simulink model "SAC_BSFC_Simulink"  (R2024b)
settings: Solver=VariableStepAuto  StartTime=0.0  StopTime=5  RelTol=1e-3
values from neighbouring files (symbols this model uses):
  BSFC = [0 0 0 0 0 0 0 0 0 0 0 0 ... (2442 elements, 37x66)]    [BSFC_LuT.mat]
  ScalerOut_range = [4.67113400e-01 3.79188137e-06 1.99107205e-09 1.76146956e-01]    [SACsim_params.m]
  ScalerOutMax = [8.17552600e-01 3.79204100e-06 1.99143300e-09 1.02194086e-01]    [SACsim_params.m]
  ScalerOutMin = [3.5043920e-01 1.5963114e-10 3.6094947e-13 -7.3952870e-02]    [SACsim_params.m]
  Tice_bp_BSFC = [0 5 10 15 20 25 30 35 40 45 50 55 ... (66 elements, 1x66)]    [BSFC_LuT.mat]
  wice_bp_BSFC = [0 13.08996939 26.1799387799 39.2699081699 52.3598775598 65.4498469498 78.5398163397 91.6297857297 104.71975512 117.80972451 130.8996939 143.98966329 ... (37 elements, 1x37)]    [BSFC_LuT.mat]
undefined symbols (not defined in the file or in its folder): a1, a2, Eng_pwr_opt_list, float32, NOx_ref, ScalerSACMax, ScalerSACMin, SoC_ref, W_list
libraries: pycoexlib x1, rllib x1
settings Model: Creator=fjcub  LastModifiedBy=fjcub

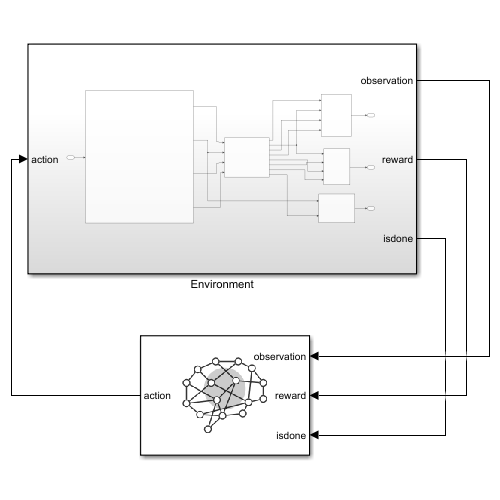
[thumbnail: Simulink's stored preview of the top-level diagram]
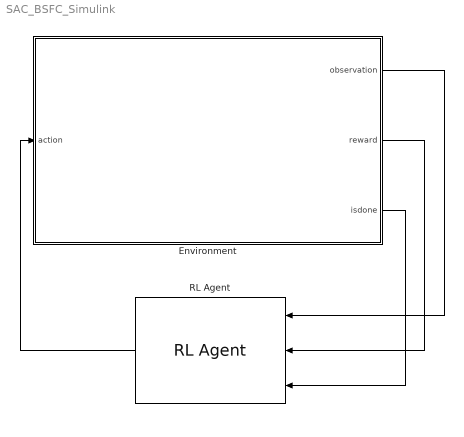
== system SAC_BSFC_Simulink ==
  Environment : Subsystem
  RL Agent : rllib/RL Agent  Agent=agent  ExternalActionAsInput=off  ProvideLastAction=off  ProvideCumRwd=off  TreatAsDirectFeedthrough=on  UseStrictObservationDataTypes=off
  wires:
  Environment/1(observation) -> RL Agent/1
  Environment/2(reward) -> RL Agent/2
  Environment/3(isdone) -> RL Agent/3
  RL Agent/1 -> Environment/1(action)

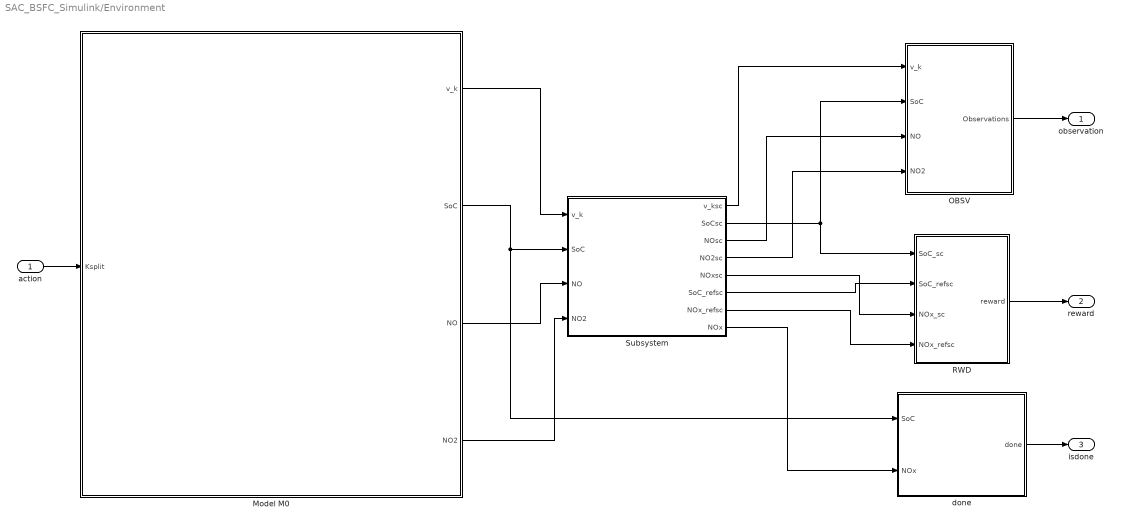
== system SAC_BSFC_Simulink/Environment ==
  action : Inport
  Model M0 : Subsystem
  OBSV : Subsystem
  RWD : Subsystem
  Subsystem : Subsystem
  done : Subsystem
  observation : Outport
  reward : Outport  Port=2
  isdone : Outport  Port=3
  wires:
  OBSV/1(Observations) -> observation/1
  action/1 -> Model M0/1(Ksplit)
  RWD/1(reward) -> reward/1
  done/1(done) -> isdone/1
  Model M0/1(v_k) -> Subsystem/1(v_k)
  Model M0/2(SoC) -> done/1(SoC), Subsystem/2(SoC)
  Model M0/3(NO) -> Subsystem/3(NO)
  Model M0/4(NO2) -> Subsystem/4(NO2)
  Subsystem/8(NOx) -> done/2(NOx)
  Subsystem/7(NOx_refsc) -> RWD/4(NOx_refsc)
  Subsystem/5(NOxsc) -> RWD/3(NOx_sc)
  Subsystem/6(SoC_refsc) -> RWD/2(SoC_refsc)
  Subsystem/2(SoCsc) -> OBSV/2(SoC), RWD/1(SoC_sc)
  Subsystem/1(v_ksc) -> OBSV/1(v_k)
  Subsystem/3(NOsc) -> OBSV/3(NO)
  Subsystem/4(NO2sc) -> OBSV/4(NO2)

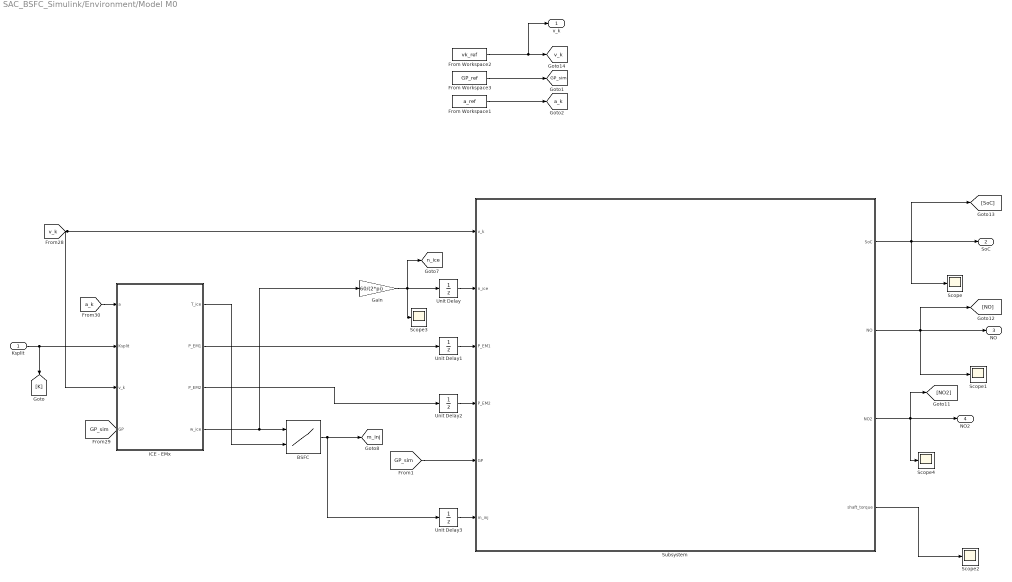
== system SAC_BSFC_Simulink/Environment/Model M0 ==
  Ksplit : Inport
  BSFC : Lookup_n-D  BreakpointsForDimension1=wice_bp_BSFC  BreakpointsForDimension2=Tice_bp_BSFC  Table=BSFC  InternalRulePriority=Speed  RndMeth=Simplest
      settings: InputPortMap=u0,u1
  From Workspace1 : FromWorkspace  VariableName=a_ref  SampleTime=1
  From Workspace2 : FromWorkspace  VariableName=vk_ref  SampleTime=1
  From Workspace3 : FromWorkspace  VariableName=GP_ref  SampleTime=1
  Gain : Gain  Gain=60/(2*pi)
  ICE - EMx : Subsystem
  Scope{,1..4} (5 alike) : Scope
  Subsystem : Subsystem
  Unit Delay{,1..3} (4 alike) : UnitDelay  SampleTime=-1  HasFrameUpgradeWarning=on
  v_k : Outport
  SoC : Outport  Port=2
  NO : Outport  Port=3
  NO2 : Outport  Port=4
  tag scope: GP_sim=global, a_k=global, m_inj=global, n_ice=global, v_k=global
  wires:
  From Workspace1/1 -> [a_k]
  From Workspace3/1 -> [GP_sim]
  From Workspace2/1 -> v_k/1, [v_k]
  Gain/1 -> Unit Delay/1, [n_ice], Scope3/1
  ICE - EMx/1(T_ice) -> BSFC/2
  Subsystem/4(shaft_torque) -> Scope2/1
  [GP_sim] -> ICE - EMx/4(GP)
  Subsystem/2(NO) -> Scope1/1, NO/1, [NO]
  [v_k] -> ICE - EMx/3(v_k), Subsystem/1(v_k)
  ICE - EMx/3(P_EM2) -> Unit Delay2/1
  Subsystem/1(SoC) -> Scope/1, SoC/1, [SoC]
  ICE - EMx/2(P_EM1) -> Unit Delay1/1
  [a_k] -> ICE - EMx/1(a)
  BSFC/1 -> Unit Delay3/1, [m_inj]
  [GP_sim] -> Subsystem/5(GP)
  ICE - EMx/4(w_ice) -> Gain/1, BSFC/1
  Ksplit/1 -> ICE - EMx/2(Ksplit), [K]
  Subsystem/3(NO2) -> [NO2], NO2/1, Scope4/1
  Unit Delay/1 -> Subsystem/2(n_ice)
  Unit Delay1/1 -> Subsystem/3(P_EM1)
  Unit Delay2/1 -> Subsystem/4(P_EM2)
  Unit Delay3/1 -> Subsystem/6(m_inj)

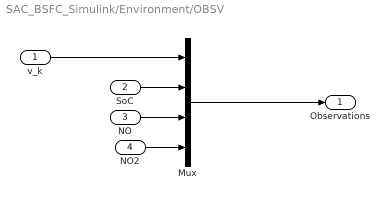
== system SAC_BSFC_Simulink/Environment/OBSV ==
  v_k : Inport
  SoC : Inport  Port=2
  NO : Inport  Port=3
  NO2 : Inport  Port=4
  Mux : Mux
  Observations : Outport
  wires:
  v_k/1 -> Mux/1
  SoC/1 -> Mux/2
  NO2/1 -> Mux/4
  NO/1 -> Mux/3
  Mux/1 -> Observations/1

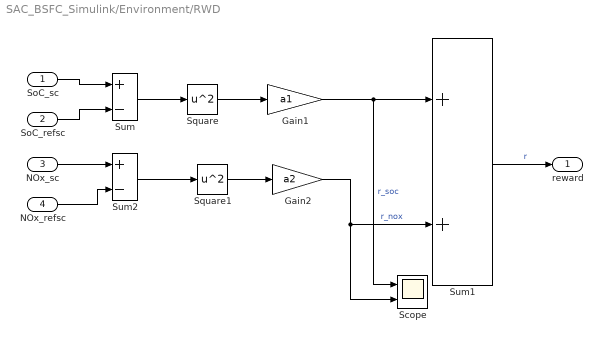
== system SAC_BSFC_Simulink/Environment/RWD ==
  SoC_sc : Inport
  SoC_refsc : Inport  Port=2
  NOx_sc : Inport  Port=3
  NOx_refsc : Inport  Port=4
  Gain1 : Gain  Gain=a1
  Gain2 : Gain  Gain=a2
  Scope : Scope  NumInputPorts=2
  Square : Math  Operator=square
  Square1 : Math  Operator=square
  Sum : Sum  Inputs=+-
  Sum1 : Sum
  Sum2 : Sum  Inputs=+-
  reward : Outport
  wires:
  Sum1/1 -> reward/1  "r"
  Sum/1 -> Square/1
  Square1/1 -> Gain2/1
  Sum2/1 -> Square1/1
  Gain1/1 -> Sum1/1, Scope/1  "r_soc"
  Gain2/1 -> Scope/2, Sum1/2  "r_nox"
  Square/1 -> Gain1/1
  SoC_sc/1 -> Sum/1
  SoC_refsc/1 -> Sum/2
  NOx_sc/1 -> Sum2/1
  NOx_refsc/1 -> Sum2/2

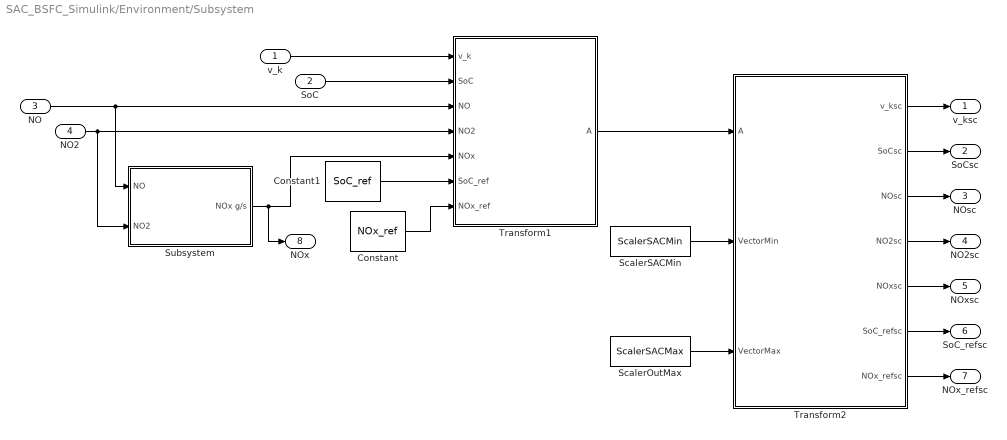
== system SAC_BSFC_Simulink/Environment/Subsystem ==
  v_k : Inport
  SoC : Inport  Port=2
  NO : Inport  Port=3
  NO2 : Inport  Port=4
  Constant : Constant  Value=NOx_ref
  Constant1 : Constant  Value=SoC_ref
  ScalerOutMax : Constant  Value=ScalerSACMax
  ScalerSACMin : Constant  Value=ScalerSACMin
  Subsystem : Subsystem
  Transform1 : MATLAB Function  TreatAsAtomicUnit=on
  Transform2 : MATLAB Function  TreatAsAtomicUnit=on
  v_ksc : Outport
  SoCsc : Outport  Port=2
  NOsc : Outport  Port=3
  NO2sc : Outport  Port=4
  NOxsc : Outport  Port=5
  SoC_refsc : Outport  Port=6
  NOx_refsc : Outport  Port=7
  NOx : Outport  Port=8
  wires:
  v_k/1 -> Transform1/1(v_k)
  SoC/1 -> Transform1/2(SoC)
  NO/1 -> Transform1/3(NO), Subsystem/1(NO)
  NO2/1 -> Subsystem/2(NO2), Transform1/4(NO2)
  Constant/1 -> Transform1/7(NOx_ref)
  Constant1/1 -> Transform1/6(SoC_ref)
  Subsystem/1(NOx g/s) -> Transform1/5(NOx), NOx/1
  Transform2/7(NOx_refsc) -> NOx_refsc/1
  Transform2/6(SoC_refsc) -> SoC_refsc/1
  Transform2/5(NOxsc) -> NOxsc/1
  Transform2/4(NO2sc) -> NO2sc/1
  Transform2/3(NOsc) -> NOsc/1
  Transform2/2(SoCsc) -> SoCsc/1
  Transform1/1(A) -> Transform2/1(A)
  ScalerSACMin/1 -> Transform2/2(VectorMin)
  ScalerOutMax/1 -> Transform2/3(VectorMax)
  Transform2/1(v_ksc) -> v_ksc/1

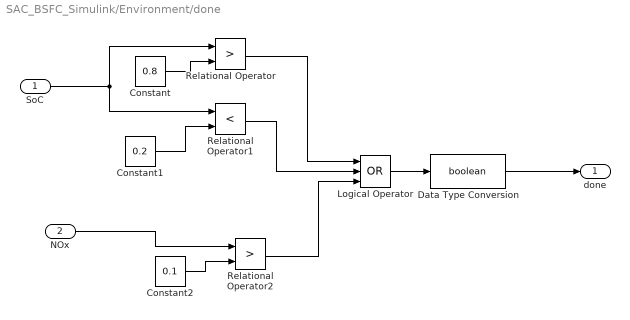
== system SAC_BSFC_Simulink/Environment/done ==
  SoC : Inport
  NOx : Inport  Port=2
  Constant : Constant  Value=0.8
  Constant1 : Constant  Value=0.2
  Constant2 : Constant  Value=0.1
  Data Type Conversion : DataTypeConversion  OutDataTypeStr=boolean  SaturateOnIntegerOverflow=off  RndMeth=Floor
  Logical Operator : Logic  Operator=OR  Inputs=3  AllPortsSameDT=off  OutDataTypeStr=boolean
  Relational Operator : RelationalOperator  Operator=>  OutDataTypeStr=boolean  RndMeth=Simplest  InputSameDT=off
  Relational Operator1 : RelationalOperator  Operator=<  OutDataTypeStr=boolean  RndMeth=Simplest  InputSameDT=off
  Relational Operator2 : RelationalOperator  Operator=>  OutDataTypeStr=boolean  RndMeth=Simplest  InputSameDT=off
  done : Outport
  wires:
  Logical Operator/1 -> Data Type Conversion/1
  Relational Operator/1 -> Logical Operator/1
  Relational Operator1/1 -> Logical Operator/2
  SoC/1 -> Relational Operator1/1, Relational Operator/1
  Constant1/1 -> Relational Operator1/2
  Constant/1 -> Relational Operator/2
  Constant2/1 -> Relational Operator2/2
  NOx/1 -> Relational Operator2/1
  Relational Operator2/1 -> Logical Operator/3
  Data Type Conversion/1 -> done/1

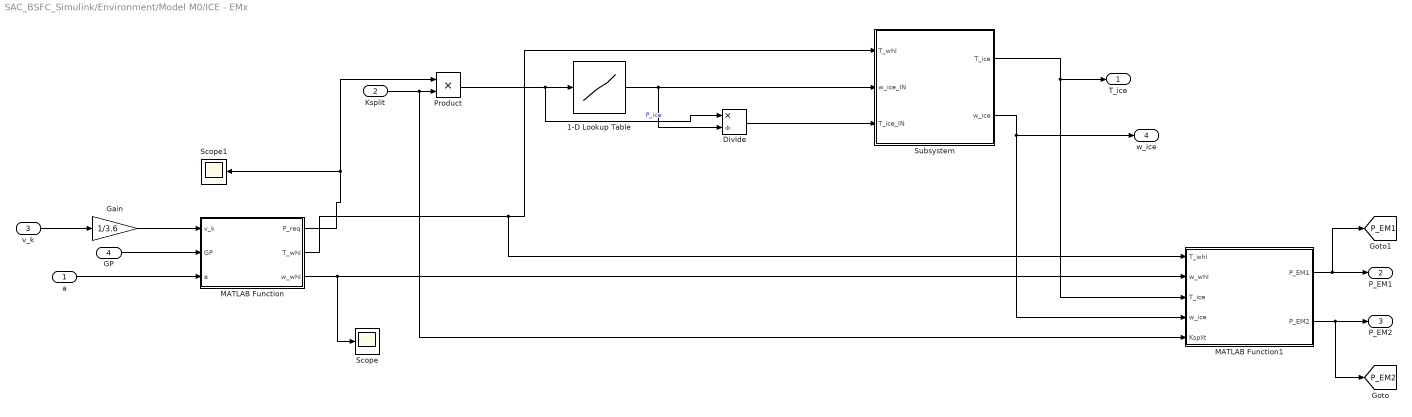
== system SAC_BSFC_Simulink/Environment/Model M0/ICE - EMx ==
  a : Inport
  Ksplit : Inport  Port=2
  v_k : Inport  Port=3
  GP : Inport  Port=4
  1-D Lookup Table : Lookup_n-D  NumberOfTableDimensions=1  BreakpointsForDimension1=Eng_pwr_opt_list  Table=W_list  InternalRulePriority=Speed  RndMeth=Simplest
  Divide : Product  Inputs=*/
  Gain : Gain  Gain=1/3.6
  MATLAB Function : MATLAB Function  TreatAsAtomicUnit=on
  MATLAB Function1 : MATLAB Function  TreatAsAtomicUnit=on
  Product : Product
  Scope : Scope
  Scope1 : Scope
  Subsystem : Subsystem
  T_ice : Outport
  P_EM1 : Outport  Port=2
  P_EM2 : Outport  Port=3
  w_ice : Outport  Port=4
  tag scope: P_EM1=global, P_EM2=global
  wires:
  MATLAB Function1/2(P_EM2) -> [P_EM2], P_EM2/1
  MATLAB Function1/1(P_EM1) -> [P_EM1], P_EM1/1
  MATLAB Function/3(w_whl) -> MATLAB Function1/2(w_whl), Scope/1
  Ksplit/1 -> MATLAB Function1/5(Ksplit), Product/2
  MATLAB Function/1(P_req) -> Product/1, Scope1/1
  GP/1 -> MATLAB Function/2(GP)
  Gain/1 -> MATLAB Function/1(v_k)
  v_k/1 -> Gain/1
  a/1 -> MATLAB Function/3(a)
  Subsystem/1(T_ice) -> T_ice/1, MATLAB Function1/3(T_ice)
  MATLAB Function/2(T_whl) -> MATLAB Function1/1(T_whl), Subsystem/1(T_whl)
  Subsystem/2(w_ice) -> MATLAB Function1/4(w_ice), w_ice/1
  Product/1 -> Divide/1, 1-D Lookup Table/1  "P_ice"
  Divide/1 -> Subsystem/3(T_ice_IN)
  1-D Lookup Table/1 -> Divide/2, Subsystem/2(w_ice_IN)

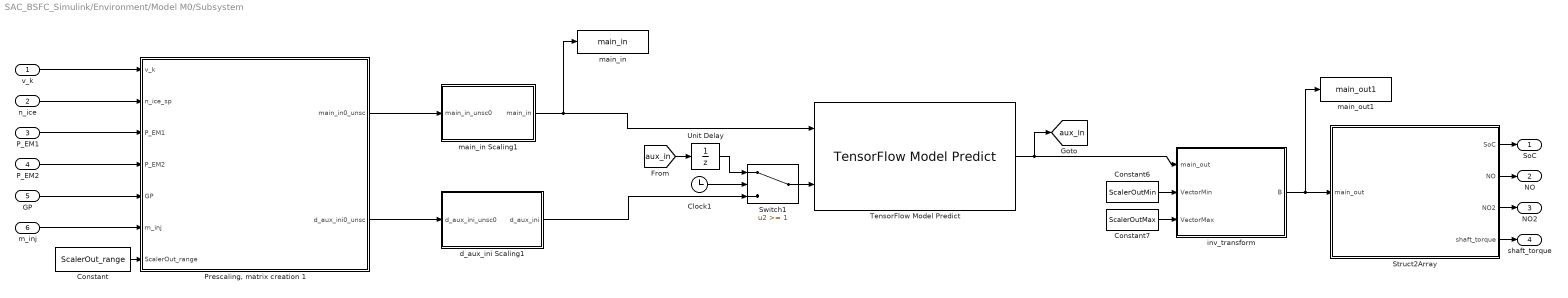
== system SAC_BSFC_Simulink/Environment/Model M0/Subsystem ==
  v_k : Inport
  n_ice : Inport  Port=2
  P_EM1 : Inport  Port=3
  P_EM2 : Inport  Port=4
  GP : Inport  Port=5
  m_inj : Inport  Port=6
  Clock1 : Clock
  Constant : Constant  Value=ScalerOut_range
  Constant6 : Constant  Value=ScalerOutMin
  Constant7 : Constant  Value=ScalerOutMax
  "Prescaling, matrix creation 1" : MATLAB Function  TreatAsAtomicUnit=on
  Struct2Array : MATLAB Function  TreatAsAtomicUnit=on
  Switch1 : Switch  Threshold=1  OutDataTypeStr=double  SaturateOnIntegerOverflow=off  InputSameDT=off
  TensorFlow Model Predict : pycoexlib/TensorFlow Model Predict  ModelFile=C:\Users\fjcub\Documents\UPC\INIREC\CORNET\Models\model.h5  InputTable={ 'main_in', 'float32', '', '3'; 'aux_in', 'float32', '', '3' }  OutputTable={ 'main_out', '', '' }  SampleTime=1  InputDatatypes=float32,float32  InputNumDims=3,3  InputPermutations=[],[]  OutputPermutations=[]  PythonCoexecutionBlockType=TensorFlowModelBlock  VariableOutputMaxSizes=[]
  Unit Delay : UnitDelay  SampleTime=-1  HasFrameUpgradeWarning=on
  d_aux_ini Scaling1 : Subsystem
  inv_transform : MATLAB Function  TreatAsAtomicUnit=on
  main_in : ToWorkspace  VariableName=main_in  SampleTime=1
  main_in Scaling1 : Subsystem
  main_out1 : ToWorkspace  VariableName=main_out1  SampleTime=1
  SoC : Outport
  NO : Outport  Port=2
  NO2 : Outport  Port=3
  shaft_torque : Outport  Port=4
  tag scope: aux_in=global
  wires:
  m_inj/1 -> "Prescaling, matrix creation 1"/6(m_inj)
  P_EM1/1 -> "Prescaling, matrix creation 1"/3(P_EM1)
  TensorFlow Model Predict/1 -> inv_transform/1(main_out), [aux_in]
  inv_transform/1(B) -> main_out1/1, Struct2Array/1(main_out)
  n_ice/1 -> "Prescaling, matrix creation 1"/2(n_ice_sp)
  Struct2Array/3(NO2) -> NO2/1
  Constant/1 -> "Prescaling, matrix creation 1"/7(ScalerOut_range)
  Constant6/1 -> inv_transform/2(VectorMin)
  P_EM2/1 -> "Prescaling, matrix creation 1"/4(P_EM2)
  "Prescaling, matrix creation 1"/1(main_in0_unsc) -> main_in Scaling1/1(main_in_unsc0)
  GP/1 -> "Prescaling, matrix creation 1"/5(GP)
  Struct2Array/2(NO) -> NO/1
  Clock1/1 -> Switch1/2
  Struct2Array/1(SoC) -> SoC/1
  Constant7/1 -> inv_transform/3(VectorMax)
  Struct2Array/4(shaft_torque) -> shaft_torque/1
  "Prescaling, matrix creation 1"/2(d_aux_ini0_unsc) -> d_aux_ini Scaling1/1(d_aux_ini_unsc0)
  main_in Scaling1/1(main_in) -> TensorFlow Model Predict/1, main_in/1
  v_k/1 -> "Prescaling, matrix creation 1"/1(v_k)
  Switch1/1 -> TensorFlow Model Predict/2
  d_aux_ini Scaling1/1(d_aux_ini) -> Switch1/3
  Unit Delay/1 -> Switch1/1
  [aux_in] -> Unit Delay/1

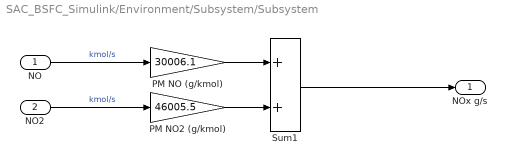
== system SAC_BSFC_Simulink/Environment/Subsystem/Subsystem ==
  NO : Inport
  NO2 : Inport  Port=2
  PM NO (g/kmol) : Gain  Gain=30006.1
  PM NO2 (g/kmol) : Gain  Gain=46005.5
  Sum1 : Sum
  NOx g/s : Outport
  wires:
  PM NO (g/kmol)/1 -> Sum1/1
  PM NO2 (g/kmol)/1 -> Sum1/2
  NO/1 -> PM NO (g/kmol)/1  "kmol/s"
  NO2/1 -> PM NO2 (g/kmol)/1  "kmol/s"
  Sum1/1 -> NOx g/s/1

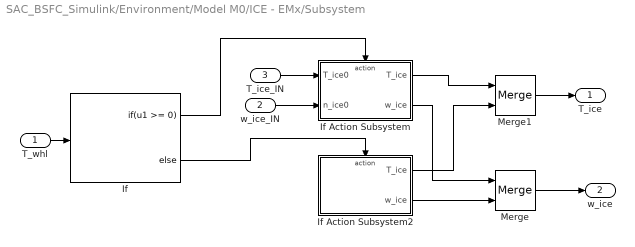
== system SAC_BSFC_Simulink/Environment/Model M0/ICE - EMx/Subsystem ==
  T_whl : Inport
  w_ice_IN : Inport  Port=2
  T_ice_IN : Inport  Port=3
  If : If  IfExpression=u1 >= 0
  If Action Subsystem : Subsystem  TreatAsAtomicUnit=on
  If Action Subsystem2 : Subsystem  TreatAsAtomicUnit=on
  Merge : Merge
  Merge1 : Merge
  T_ice : Outport
  w_ice : Outport  Port=2
  wires:
  T_whl/1 -> If/1
  If/1 -> If Action Subsystem/Action
  If/2 -> If Action Subsystem2/Action
  T_ice_IN/1 -> If Action Subsystem/1(T_ice0)
  w_ice_IN/1 -> If Action Subsystem/2(n_ice0)
  If Action Subsystem/1(T_ice) -> Merge1/1
  If Action Subsystem2/1(T_ice) -> Merge1/2
  If Action Subsystem/2(w_ice) -> Merge/1
  If Action Subsystem2/2(w_ice) -> Merge/2
  Merge/1 -> w_ice/1
  Merge1/1 -> T_ice/1

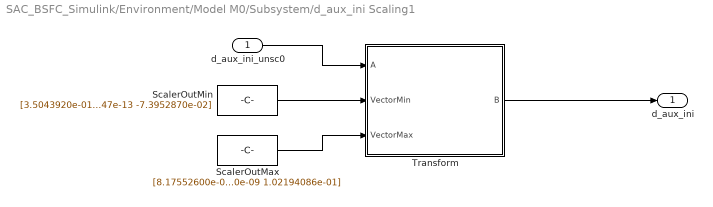
== system SAC_BSFC_Simulink/Environment/Model M0/Subsystem/d_aux_ini Scaling1 ==
  d_aux_ini_unsc0 : Inport
  ScalerOutMax : Constant  Value=[8.17552600e-01 3.79204100e-06 1.99143300e-09 1.02194086e-01]
  ScalerOutMin : Constant  Value=[3.5043920e-01 1.5963114e-10 3.6094947e-13 -7.3952870e-02]
  Transform : MATLAB Function  TreatAsAtomicUnit=on
  d_aux_ini : Outport
  wires:
  d_aux_ini_unsc0/1 -> Transform/1(A)
  ScalerOutMin/1 -> Transform/2(VectorMin)
  ScalerOutMax/1 -> Transform/3(VectorMax)
  Transform/1(B) -> d_aux_ini/1

== system SAC_BSFC_Simulink/Environment/Model M0/Subsystem/main_in Scaling1 ==
  main_in_unsc0 : Inport
  ScalerInMax : Constant  Value=[1.5060300e+02; 2.8380360e+03; 8.5859970e+00; 5.1123200e+01; 4.4160643e+00; 1.2493309e+00]
  ScalerInMin : Constant  Value="[-5.9009795; 1287.4781; -54.729496;  -3.403699; -4.377029; 0.]"
  Transform : MATLAB Function  TreatAsAtomicUnit=on
  main_in : Outport
  wires:
  Transform/1(B) -> main_in/1
  main_in_unsc0/1 -> Transform/1(A)
  ScalerInMax/1 -> Transform/3(VectorMax)
  ScalerInMin/1 -> Transform/2(VectorMin)

== system SAC_BSFC_Simulink/Environment/Model M0/ICE - EMx/Subsystem/If Action Subsystem ==
  T_ice0 : Inport
  n_ice0 : Inport  Port=2
  Action Port : ActionPort  ActionPortLabel=if(u1 >= 0)
  T_ice : Outport
  w_ice : Outport  Port=2
  wires:
  T_ice0/1 -> T_ice/1
  n_ice0/1 -> w_ice/1

== system SAC_BSFC_Simulink/Environment/Model M0/ICE - EMx/Subsystem/If Action Subsystem2 ==
  Action Port : ActionPort  ActionPortLabel=else
  Constant : Constant  Value=0  SampleTime=1
  Constant1 : Constant  Value=0  SampleTime=1
  T_ice : Outport
  w_ice : Outport  Port=2
  wires:
  Constant/1 -> T_ice/1
  Constant1/1 -> w_ice/1

== matlab function SAC_BSFC_Simulink/Environment/Model M0/Subsystem/main_in Scaling1/Transform ==
  data: A input; B output; VectorMin input; VectorMax input
function B = transform(A,VectorMin,VectorMax)
max=1;
min=-1;
B=ones(1,1,length(A));
    for i=1:1:length(A)
        X_std=(A(1,1,i)-VectorMin(i))/(VectorMax(i)-VectorMin(i));
        X_scaled=X_std*(max-min)+min;
        B(1,1,i)=X_scaled;
    end
end

== matlab function SAC_BSFC_Simulink/Environment/Model M0/Subsystem/inv_transform ==
  data: main_out input; B output; VectorMin input; VectorMax input
function B = inv_transform(main_out,VectorMin,VectorMax)
A=ones(1,1,4);
maxbound=1;
minbound=-1;
A(:,:,:)=main_out(:,:,:);
B=ones(1,1,4);
    for i=1:1:length(A)
        X_std=(A(1,1,i)-minbound)/(maxbound-minbound);
        X_scaled=X_std*(VectorMax(i)-VectorMin(i))+VectorMin(i);
        B(1,1,i)=X_scaled;
    end
end

== matlab function SAC_BSFC_Simulink/Environment/Model M0/Subsystem/Prescaling, matrix creation 1 ==
  data: v_k input; main_in0_unsc output; n_ice_sp input; P_EM1 input; P_EM2 input; GP input; m_inj input; d_aux_ini0_unsc output; ScalerOut_range input
function [main_in0_unsc,d_aux_ini0_unsc]= prescaler(v_k,n_ice_sp,P_EM1, P_EM2, GP, m_inj,ScalerOut_range)


main_in=ones(1,1,6);
main_in(1,1,1) = v_k; %Velocity_kph
main_in(1,1,2) = n_ice_sp; %Engine_Speed_RPM similar to set point
main_in(1,1,3) = P_EM1;  %EM1 Power similar to set point
main_in(1,1,4) = P_EM2;  %EM2 Power similar to set point
main_in(1,1,5) = GP; %Grade in percentage
main_in(1,1,6) = m_inj; %Injection mass similar to set point

d_aux_ini = ones(1,1,4);
for i=1:1:4
    d_aux_ini(1,1,i)=ScalerOut_range(i)/2;
end

d_aux_ini0_unsc=d_aux_ini(1,1,:); 
main_in0_unsc=main_in(1,1,:); %El output se corresponde con el que da main_in[0] en Python

%%PYTHON CODE
% # Scaling input main
% main_in[0] = scalerIn.transform(main_in[0])
% v = model.predict([main_in, d_aux_ini], batch_size=1, steps=1)
% 
% # Transforming scaled values to orignal space
% vo = scalerOut.inverse_transform(v[0])
% dataY.append(vo)

== matlab function SAC_BSFC_Simulink/Environment/Model M0/Subsystem/Struct2Array ==
  data: SoC output; NO output; NO2 output; shaft_torque output; main_out input
function [SoC, NO, NO2, shaft_torque] = getvars(main_out)
SoC=main_out(1,1,1);
NO=main_out(1,1,2);
NO2=main_out(1,1,3);
shaft_torque=main_out(1,1,4);
end

== matlab function SAC_BSFC_Simulink/Environment/Model M0/Subsystem/d_aux_ini Scaling1/Transform ==
  data: A input; B output; VectorMin input; VectorMax input
function B = transform(A,VectorMin,VectorMax)
    max=1;
    min=-1;
    B=ones(1,1,length(A));
    for i=1:1:length(A)
        X_std=(A(1,1,i)-VectorMin(i))/(VectorMax(i)-VectorMin(i));
        X_scaled=X_std*(max-min)+min;
        B(1,1,i)=X_scaled;
    end
end

== matlab function SAC_BSFC_Simulink/Environment/Model M0/ICE - EMx/MATLAB Function ==
  data: P_req output; v_k input; T_whl output; GP input; a input; w_whl output
function [P_req, T_whl, w_whl] = CalcTorque(v_k,GP,a)
g = 9.81;                            %Gravity, m/s^2
m= 1750;                         % Vehicle mass, Kg
f = 0.01;                            % Rolling coefficient, N·m
C_d = 0.26;
A = 2.33;
R_roll = 0.3;
v=v_k/3.6;

theta=atan(GP/100);
w_whl=v_k/R_roll;

T_whl=R_roll*(m*a+m*g*f*cos(theta)+m*g*sin(theta)+(C_d*A*v^2)/21.15);
P_req=T_whl*w_whl;

== matlab function SAC_BSFC_Simulink/Environment/Model M0/ICE - EMx/MATLAB Function1 ==
  data: T_whl input; P_EM1 output; w_whl input; T_ice input; w_ice input; P_EM2 output; Ksplit input
function [P_EM1, P_EM2]=EMx_Power(T_whl, w_whl, T_ice, w_ice,Ksplit)
     k1=1.92;
     k2=2.6;
     kf=4.1;

     if Ksplit==0;
        w_ice=0;
        w_EM1=(k1+1)*kf*w_whl;
        w_EM2=-k2*kf*w_whl;
        T_EM2=-T_whl/(k2*kf);
        T_EM1=0;
     else
         T_EM2 = 1 / (k1 + k2 + 1) * (T_whl * k1 / kf - (k1 + 1) * T_ice); %Formulas from the paper, steady-state eCVT2 with EM1 as speeder
         T_EM1 = 1 / k1 * T_ice + (k2 + 1) / k1 * T_EM2;
         w_C1R2 = kf * w_whl;
         w_EM1 = (k1 + 1) * w_C1R2 - k1 * w_ice;
         w_EM2 = (k1 + k2 + 1) / k1 * w_C1R2 - (k2 + 1) / k1 * w_C1R2;
     end
     P_EM1 = w_EM1 * T_EM1 * 0.001;
     P_EM2 = w_EM2 * T_EM2 * 0.001;
end

== matlab function SAC_BSFC_Simulink/Environment/Subsystem/Transform1 ==
  data: v_k input; A output; SoC input; NO input; NO2 input; NOx input; SoC_ref input; NOx_ref input
function A = matrixmaker(v_k, SoC, NO, NO2, NOx, SoC_ref, NOx_ref)

A=ones(1,7);
A(1,1)=v_k;
A(1,2)=SoC;
A(1,3)=NO;
A(1,4)=NO2;
A(1,5)=NOx;
A(1,6)=SoC_ref;
A(1,7)=NOx_ref;

end

== matlab function SAC_BSFC_Simulink/Environment/Subsystem/Transform2 ==
  data: A input; v_ksc output; VectorMin input; VectorMax input; SoCsc output; NOsc output; NO2sc output; NOxsc output; SoC_refsc output; NOx_refsc output
function [v_ksc,SoCsc,NOsc,NO2sc,NOxsc,SoC_refsc,NOx_refsc] = transform(A,VectorMin,VectorMax)
    max=1;
    min=0;
    B=ones(1,length(A));
    for i=1:1:length(A)
        X_std=(A(1,i)-VectorMin(i))/(VectorMax(i)-VectorMin(i));
        X_scaled=X_std*(max-min)+min;
        B(1,i)=X_scaled;
    end
    
    v_ksc=B(1,1);
    SoCsc=B(1,2);
    NOsc=B(1,3);
    NO2sc=B(1,4);
    NOxsc=B(1,5);
    SoC_refsc=B(1,6);
    NOx_refsc=B(1,7);
end
